simulink model "systemIO"  (R2018a)
settings: Solver=VariableStepAuto  StartTime=0.0  StopTime=10.0  RelTol=1e-3
libraries: arduinolib x4, simulink x2
settings Model: Creator=thanhdo  LastModifiedBy=thanhdo

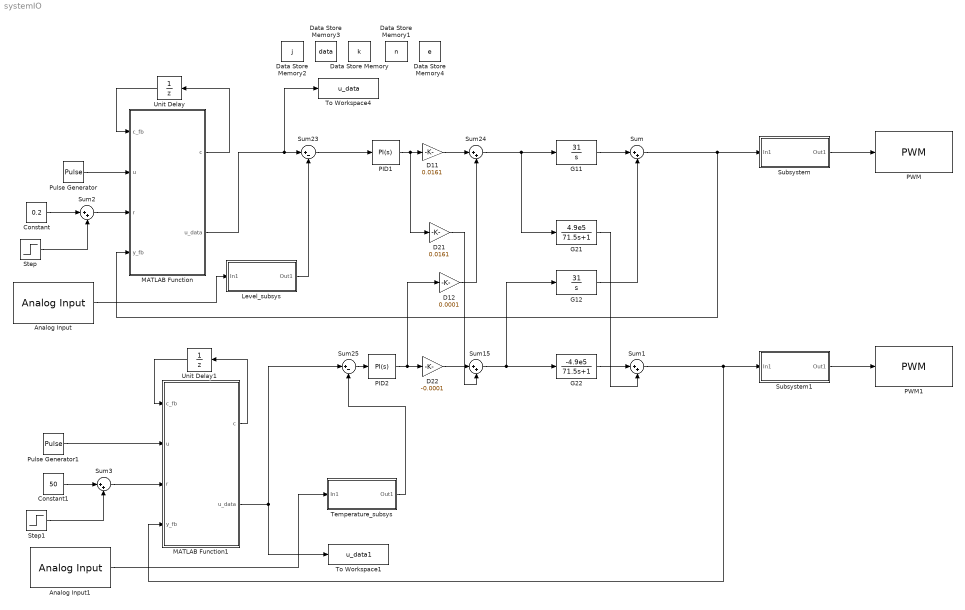
== system systemIO ==
  Analog Input : arduinolib/Analog Input  pinNumber=4  ReadResultsOnly=off  ConversionTriggerSource=Software  ExternalTriggerType=uint32(0)  OutputDataType=uint16  EnableConversionCompleteNotify=off  EnableOuputStatus=off  SampleTime=1  blockPlatform=arduino
  Analog Input1 : arduinolib/Analog Input  pinNumber=5  ReadResultsOnly=off  ConversionTriggerSource=Software  ExternalTriggerType=uint32(0)  OutputDataType=uint16  EnableConversionCompleteNotify=off  EnableOuputStatus=off  SampleTime=1  blockPlatform=arduino
  Constant : Constant  Value=0.2
  Constant1 : Constant  Value=50
  D11 : Gain  Gain=0.0161
  D12 : Gain  Gain=0.0001
  D21 : Gain  Gain=0.0161
  D22 : Gain  Gain=-0.0001
  Data Store Memory : DataStoreMemory  DataStoreName=k  ReadBeforeWriteMsg=warning  WriteAfterWriteMsg=warning  WriteAfterReadMsg=warning  ShowAdditionalParam=off  OutDataTypeStr=double
  Data Store Memory1 : DataStoreMemory  DataStoreName=n  ReadBeforeWriteMsg=warning  WriteAfterWriteMsg=warning  WriteAfterReadMsg=warning  ShowAdditionalParam=off  OutDataTypeStr=double
  Data Store Memory2 : DataStoreMemory  DataStoreName=j  ReadBeforeWriteMsg=warning  WriteAfterWriteMsg=warning  WriteAfterReadMsg=warning  ShowAdditionalParam=off  OutDataTypeStr=double
  Data Store Memory3 : DataStoreMemory  DataStoreName=data  ReadBeforeWriteMsg=warning  WriteAfterWriteMsg=warning  WriteAfterReadMsg=warning  ShowAdditionalParam=off  OutDataTypeStr=double  Dimensions=[1 120]
  Data Store Memory4 : DataStoreMemory  DataStoreName=e  ReadBeforeWriteMsg=warning  WriteAfterWriteMsg=warning  WriteAfterReadMsg=warning  ShowAdditionalParam=off  OutDataTypeStr=double  Dimensions=[1 120]
  G11 : TransferFcn  Numerator=[31]  Denominator=[1 0]
  "G12 " : TransferFcn  Numerator=[31]  Denominator=[1 0]
  G21 : TransferFcn  Numerator=[4.9e5]  Denominator=[71.5 1]
  G22 : TransferFcn  Numerator=[-4.9e5]  Denominator=[71.5 1]
  Level_subsys : Subsystem
  MATLAB Function : MATLAB Function  TreatAsAtomicUnit=on
  MATLAB Function1 : MATLAB Function  TreatAsAtomicUnit=on
  PID1 : simulink/Continuous/PID Controller  Controller=PI  TimeDomain=Continuous-time  SampleTime=-1  IntegratorMethod=Forward Euler  FilterMethod=Forward Euler  Form=Parallel  UseFilter=on  ControllerParametersSource=internal  P=3  I=0.1  D=0  N=100  InitialConditionSource=internal  InitialConditionForIntegrator=0  InitialConditionForFilter=0  ExternalReset=none  LimitOutput=off  UpperSaturationLimit=inf  LowerSaturationLimit=-inf  LinearizeAsGain=on  AntiWindupMode=none  Kb=1  TrackingMode=off  Kt=1  PParamMin=[]  PParamMax=[]  IParamMin=[]  IParamMax=[]  DParamMin=[]  DParamMax=[]  NParamMin=[]  NParamMax=[]  KbParamMin=[]  KbParamMax=[]  KtParamMin=[]  KtParamMax=[]  POutMin=[]  POutMax=[]  IOutMin=[]  IOutMax=[]  DOutMin=[]  DOutMax=[]  NOutMin=[]  NOutMax=[]  KbOutMin=[]  KbOutMax=[]  KtOutMin=[]  KtOutMax=[]  IntegratorOutMin=[]  IntegratorOutMax=[]  FilterOutMin=[]  FilterOutMax=[]  SumOutMin=[]  SumOutMax=[]  SumI1OutMin=[]  SumI1OutMax=[]  SumI2OutMin=[]  SumI2OutMax=[]  SumI3OutMin=[]  SumI3OutMax=[]  SumDOutMin=[]  SumDOutMax=[]  SaturationOutMin=[]  SaturationOutMax=[]  IntegratorContinuousStateAttributes=''  IntegratorStateMustResolveToSignalObject=off  IntegratorRTWStateStorageClass=Auto  FilterContinuousStateAttributes=''  FilterStateMustResolveToSignalObject=off  FilterRTWStateStorageClass=Auto  DifferentiatorICPrevScaledInput=0  DifferentiatorOutMin=[]  DifferentiatorOutMax=[]  FilterDiffOutCoefMin=[]  FilterDiffOutCoefMax=[]  SumDenOutMin=[]  SumDenOutMax=[]  SumNumOutMin=[]  SumNumOutMax=[]  ReciprocalOutMin=[]  ReciprocalOutMax=[]  DivideOutMin=[]  DivideOutMax=[]  TunerSelectOption=Transfer Function Based (PID Tuner App)
  PID2 : simulink/Continuous/PID Controller  Controller=PI  TimeDomain=Continuous-time  SampleTime=-1  IntegratorMethod=Forward Euler  FilterMethod=Forward Euler  Form=Parallel  UseFilter=on  ControllerParametersSource=internal  P=1  I=0.03  D=0  N=100  InitialConditionSource=internal  InitialConditionForIntegrator=0  InitialConditionForFilter=0  ExternalReset=none  LimitOutput=off  UpperSaturationLimit=inf  LowerSaturationLimit=-inf  LinearizeAsGain=on  AntiWindupMode=none  Kb=1  TrackingMode=off  Kt=1  PParamMin=[]  PParamMax=[]  IParamMin=[]  IParamMax=[]  DParamMin=[]  DParamMax=[]  NParamMin=[]  NParamMax=[]  KbParamMin=[]  KbParamMax=[]  KtParamMin=[]  KtParamMax=[]  POutMin=[]  POutMax=[]  IOutMin=[]  IOutMax=[]  DOutMin=[]  DOutMax=[]  NOutMin=[]  NOutMax=[]  KbOutMin=[]  KbOutMax=[]  KtOutMin=[]  KtOutMax=[]  IntegratorOutMin=[]  IntegratorOutMax=[]  FilterOutMin=[]  FilterOutMax=[]  SumOutMin=[]  SumOutMax=[]  SumI1OutMin=[]  SumI1OutMax=[]  SumI2OutMin=[]  SumI2OutMax=[]  SumI3OutMin=[]  SumI3OutMax=[]  SumDOutMin=[]  SumDOutMax=[]  SaturationOutMin=[]  SaturationOutMax=[]  IntegratorContinuousStateAttributes=''  IntegratorStateMustResolveToSignalObject=off  IntegratorRTWStateStorageClass=Auto  FilterContinuousStateAttributes=''  FilterStateMustResolveToSignalObject=off  FilterRTWStateStorageClass=Auto  DifferentiatorICPrevScaledInput=0  DifferentiatorOutMin=[]  DifferentiatorOutMax=[]  FilterDiffOutCoefMin=[]  FilterDiffOutCoefMax=[]  SumDenOutMin=[]  SumDenOutMax=[]  SumNumOutMin=[]  SumNumOutMax=[]  ReciprocalOutMin=[]  ReciprocalOutMax=[]  DivideOutMin=[]  DivideOutMax=[]  TunerSelectOption=Transfer Function Based (PID Tuner App)
  PWM : arduinolib/PWM  pinNumber=5  EnableInputFrequency=off  InitialFrequency=2000  InitialDutyCycle=0  NotificationType=None  blockPlatform=arduino
  PWM1 : arduinolib/PWM  pinNumber=7  EnableInputFrequency=off  InitialFrequency=2000  InitialDutyCycle=0  NotificationType=None  blockPlatform=arduino
  Pulse Generator : DiscretePulseGenerator  PulseType=Time based  Period=0.2  PulseWidth=50  PhaseDelay=0.1
  Pulse Generator1 : DiscretePulseGenerator  PulseType=Time based  Period=0.2  PulseWidth=50  PhaseDelay=0.1
  Step : Step  Time=30  After=0.05  SampleTime=0
  Step1 : Step  Time=50  After=10  SampleTime=0
  Subsystem : Subsystem
  Subsystem1 : Subsystem
  Sum{,1..3,15,24} (6 alike) : Sum  Inputs=|++
  Sum23 : Sum  Inputs=|+-
  Sum25 : Sum  Inputs=|+-
  Temperature_subsys : Subsystem
  To Workspace1 : ToWorkspace  VariableName=u_data1  SampleTime=-1
      settings: Save2DSignal=2-D array (concatenate along first dimension)
  To Workspace4 : ToWorkspace  VariableName=u_data  SampleTime=-1
      settings: Save2DSignal=2-D array (concatenate along first dimension)
  Unit Delay : UnitDelay  InitialCondition=1  SampleTime=-1
  Unit Delay1 : UnitDelay  InitialCondition=1  SampleTime=-1
  wires:
  Step1/1 -> Sum3/2
  PID2/1 -> D12/1, D22/1
  Sum2/1 -> MATLAB Function/3(r)
  Constant/1 -> Sum2/1
  Sum3/1 -> MATLAB Function1/3(r)
  Pulse Generator1/1 -> MATLAB Function1/2(u)
  Sum1/1 -> Subsystem1/1(In1), MATLAB Function1/4(y_fb)
  Step/1 -> Sum2/2
  Unit Delay/1 -> MATLAB Function/1(c_fb)
  Constant1/1 -> Sum3/1
  MATLAB Function/2(u_data) -> To Workspace4/1, Sum23/1
  Sum/1 -> Subsystem/1(In1), MATLAB Function/4(y_fb)
  MATLAB Function1/1(c) -> Unit Delay1/1
  MATLAB Function1/2(u_data) -> To Workspace1/1, Sum25/1
  Sum15/1 -> "G12 "/1, G22/1
  Unit Delay1/1 -> MATLAB Function1/1(c_fb)
  MATLAB Function/1(c) -> Unit Delay/1
  PID1/1 -> D11/1, D21/1
  G11/1 -> Sum/1
  Pulse Generator/1 -> MATLAB Function/2(u)
  G22/1 -> Sum1/1
  G21/1 -> Sum1/2
  Sum24/1 -> G21/1, G11/1
  "G12 "/1 -> Sum/2
  Sum23/1 -> PID1/1
  D12/1 -> Sum24/2
  D21/1 -> Sum15/2
  D22/1 -> Sum15/1
  Sum25/1 -> PID2/1
  D11/1 -> Sum24/1
  Level_subsys/1(Out1) -> Sum23/2
  Analog Input/1 -> Level_subsys/1(In1)
  Temperature_subsys/1(Out1) -> Sum25/2
  Analog Input1/1 -> Temperature_subsys/1(In1)
  Subsystem/1(Out1) -> PWM/1
  Subsystem1/1(Out1) -> PWM1/1

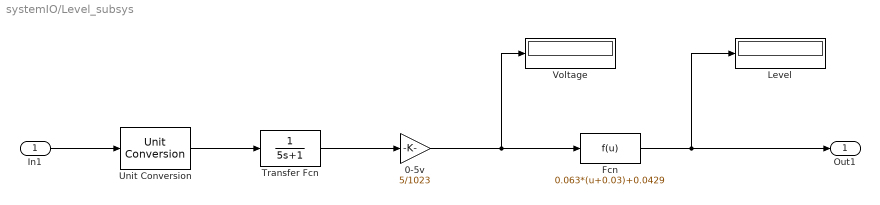
== system systemIO/Level_subsys ==
  In1 : Inport
  0-5v : Gain  Gain=5/1023
  Fcn : Fcn  Expr=0.063*(u+0.03)+0.0429
  Level : Display
  Transfer Fcn : TransferFcn  Denominator=[5 1]
  Unit Conversion : UnitConversion
  Voltage : Display
  Out1 : Outport
  wires:
  Unit Conversion/1 -> Transfer Fcn/1
  Transfer Fcn/1 -> 0-5v/1
  Fcn/1 -> Out1/1, Level/1
  0-5v/1 -> Voltage/1, Fcn/1
  In1/1 -> Unit Conversion/1

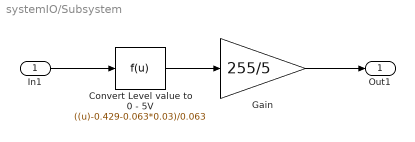
== system systemIO/Subsystem ==
  In1 : Inport
  "Convert Level value to 0 - 5V " : Fcn  Expr=((u)-0.429-0.063*0.03)/0.063
  Gain : Gain  Gain=255/5
  Out1 : Outport
  wires:
  "Convert Level value to 0 - 5V "/1 -> Gain/1
  In1/1 -> "Convert Level value to 0 - 5V "/1
  Gain/1 -> Out1/1

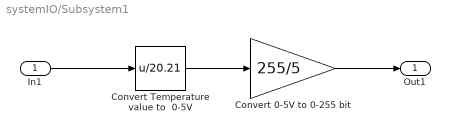
== system systemIO/Subsystem1 ==
  In1 : Inport
  "Convert 0-5V to 0-255 bit " : Gain  Gain=255/5
  Convert Temperature value to  0-5V : Fcn  Expr=u/20.21
  Out1 : Outport
  wires:
  Convert Temperature value to  0-5V/1 -> "Convert 0-5V to 0-255 bit "/1
  In1/1 -> Convert Temperature value to  0-5V/1
  "Convert 0-5V to 0-255 bit "/1 -> Out1/1

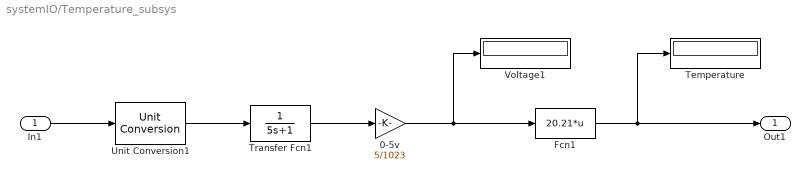
== system systemIO/Temperature_subsys ==
  In1 : Inport
  0-5v : Gain  Gain=5/1023
  Fcn1 : Fcn  Expr=20.21*u
  Temperature : Display
  Transfer Fcn1 : TransferFcn  Denominator=[5 1]
  Unit Conversion1 : UnitConversion
  Voltage1 : Display
  Out1 : Outport
  wires:
  Unit Conversion1/1 -> Transfer Fcn1/1
  0-5v/1 -> Fcn1/1, Voltage1/1
  Fcn1/1 -> Out1/1, Temperature/1
  Transfer Fcn1/1 -> 0-5v/1
  In1/1 -> Unit Conversion1/1

== matlab function systemIO/MATLAB Function1 ==
  settings: updateMethod=DISCRETE
  data: c_fb input; u input; c output; k data_store_memory; n data_store_memory; j data_store_memory; data data_store_memory; e data_store_memory; r input; y_fb input; u_data output
function [c, u_data] = fcn(c_fb, u, r, y_fb)
c=u;

t=c_fb;y_1=0;
global k n j data e

if t~=u
    k=k+1;
    if k==1
        n=n+1;
    end
end
if rem(k,120)==1 && k>120
    n=n+1; % number of Iterative
end

if n==1 
    j=k; % j index 
elseif n>1
    j=k-(n-1)*120;
end


if n==1
    if j==1
        e(j)=r-y_1;% error e=r-y_fb
    else
        e(j)=r-y_fb;% error e=r-y_fb
    end
    data(j)=r+0.1*e(j); %correction formula u(i)=u(i)+k*r with iterative n=1 replace u(i)=> r
elseif n>=2 
    e(j)=r-y_fb;
    data(j)=data(j)+0.1*e(j); 
end

u_data=data(j); % send u_dk to plant

== matlab function systemIO/MATLAB Function ==
  settings: updateMethod=DISCRETE
  data: c_fb input; u input; c output; k data_store_memory; n data_store_memory; j data_store_memory; data data_store_memory; e data_store_memory; r input; y_fb input; u_data output
function [c, u_data] = fcn(c_fb, u, r, y_fb)
c=u;

t=c_fb;y_1=0;
global k n j data e

if t~=u
    k=k+1;
    if k==1
        n=n+1;
    end
end
if rem(k,120)==1 && k>120
    n=n+1; % number of Iterative
end

if n==1 
    j=k; % j index 
elseif n>1
    j=k-(n-1)*120;
end


if n==1
    if j==1
        e(j)=r-y_1;% error e=r-y_fb
    else
        e(j)=r-y_fb;% error e=r-y_fb
    end
    data(j)=r+0.05*e(j); %correction formula u(i)=u(i)+k*r with iterative n=1 replace u(i)=> r
elseif n>=2 
    e(j)=r-y_fb;
    data(j)=data(j)+0.05*e(j); 
end

u_data=data(j); % send u_dk to plant
